simulink model "obserwator"  (R2021a)
settings: Solver=VariableStepAuto  StartTime=0.0  StopTime=10.0  RelTol=1e-3
values from neighbouring files (symbols this model uses):
  L1 = L(1)    [liczenie_l_num.m]    (also in skrypt_k_i_l.m)
  L2 = L(2)    [liczenie_l_num.m]    (also in skrypt_k_i_l.m)
  L3 = L(3)    [liczenie_l_num.m]    (also in skrypt_k_i_l.m)
settings Model: Creator=ADMIN  LastModifiedBy=ADMIN

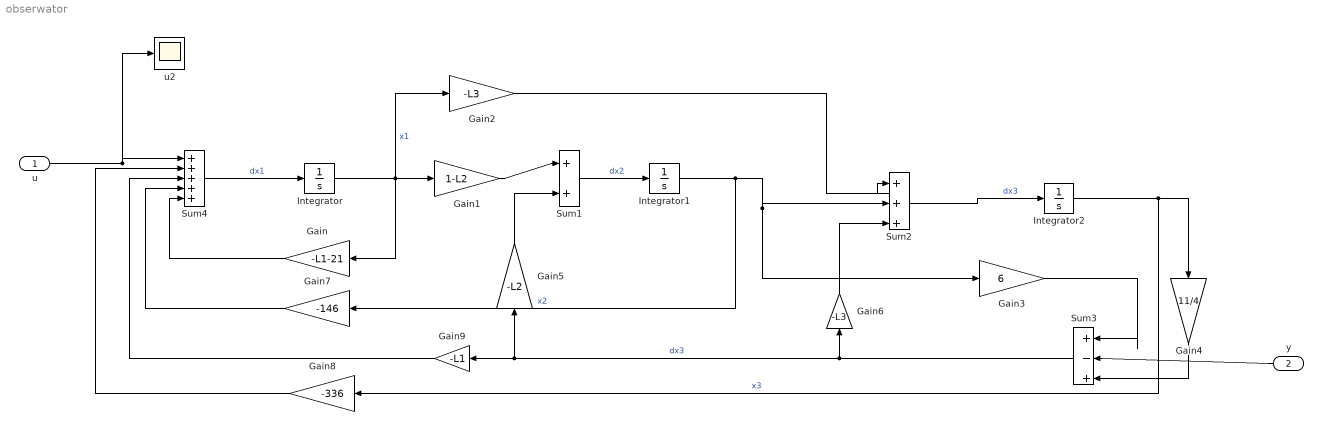
== system obserwator ==
  u : Inport
  y : Inport  Port=2
  Gain : Gain  Gain=-L1-21
  Gain1 : Gain  Gain=1-L2
  Gain2 : Gain  Gain=-L3
  Gain3 : Gain  Gain=6
  Gain4 : Gain  Gain=11/4
  Gain5 : Gain  Gain=-L2
  Gain6 : Gain  Gain=-L3
  Gain7 : Gain  Gain=-146
  Gain8 : Gain  Gain=-336
  Gain9 : Gain  Gain=-L1
  Integrator : Integrator
  Integrator1 : Integrator
  Integrator2 : Integrator
  Sum1 : Sum  Inputs=|++
  Sum2 : Sum  Inputs=|+++
  Sum3 : Sum  Inputs=|+-+
  Sum4 : Sum  Inputs=|+++++
  u2 : Scope
  wires:
  u/1 -> u2/1, Sum4/1
  Sum4/1 -> Integrator/1  "dx1"
  Integrator/1 -> Gain2/1, Gain1/1, Gain/1  "x1"
  Sum1/1 -> Integrator1/1  "dx2"
  Integrator1/1 -> Gain7/1, Sum2/2, Gain3/1  "x2"
  Sum2/1 -> Integrator2/1  "dx3"
  Integrator2/1 -> Gain8/1, Gain4/1  "x3"
  Gain/1 -> Sum4/5
  Gain1/1 -> Sum1/1
  Gain2/1 -> Sum2/1
  y/1 -> Sum3/2
  Gain3/1 -> Sum3/1
  Gain4/1 -> Sum3/3
  Sum3/1 -> Gain6/1, Gain9/1, Gain5/1  "dx3"
  Gain5/1 -> Sum1/2
  Gain6/1 -> Sum2/3
  Gain7/1 -> Sum4/4
  Gain8/1 -> Sum4/2
  Gain9/1 -> Sum4/3
